simulink model "Nils_Bestehorn_WS19_modell"  (R2021b)
settings: Solver=FixedStepAuto  StartTime=0.0  StopTime=1  FixedStep=0.001  RelTol=1e-3
values from neighbouring files (symbols this model uses):
  c = 50    [Nils_Bestehorn_WS19_mfile.m]
  d = 0.05    [Nils_Bestehorn_WS19_mfile.m]
  dL = 5*exp(-6)    [Nils_Bestehorn_WS19_mfile.m]
  dM = 1.0*exp(-5)    [Nils_Bestehorn_WS19_mfile.m]
  JL = 2*exp(-5)    [Nils_Bestehorn_WS19_mfile.m]
  JM = 0.125*exp(-5)    [Nils_Bestehorn_WS19_mfile.m]
  LM = 1.0*exp(-3)    [Nils_Bestehorn_WS19_mfile.m]
  ML = 0.25    [Nils_Bestehorn_WS19_mfile.m]
  omegaL = 2.6*exp(-2)    [Nils_Bestehorn_WS19_mfile.m]
  omegaM = 0.1125    [Nils_Bestehorn_WS19_mfile.m]
  rL = 50*10^(-3)    (= 0.05)    [Nils_Bestehorn_WS19_mfile.m]
  RM = 1.5    [Nils_Bestehorn_WS19_mfile.m]
  rM = 25*10^(-3)    (= 0.025)    [Nils_Bestehorn_WS19_mfile.m]
  Uq = 24    [Nils_Bestehorn_WS19_mfile.m]
settings Model: Creator=nilsb  LastModifiedBy=nilsb

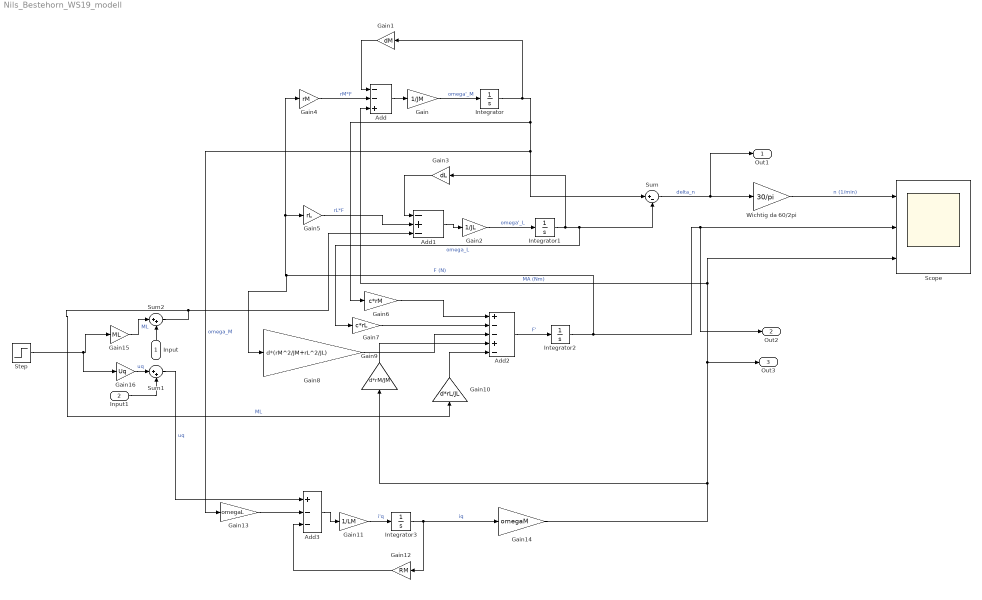
== system Nils_Bestehorn_WS19_modell ==
  Input : Inport
  Input1 : Inport  Port=2
  Add : Sum  Inputs=--+
  Add1 : Sum  Inputs=-+-
  Add2 : Sum  Inputs=+--+-
  Add3 : Sum  Inputs=+--
  Gain : Gain  Gain=1/JM
  Gain1 : Gain  Gain=dM
  Gain10 : Gain  Gain=d*rL/JL
  Gain11 : Gain  Gain=1/LM
  Gain12 : Gain  Gain=RM
  Gain13 : Gain  Gain=omegaL
  Gain14 : Gain  Gain=omegaM
  Gain15 : Gain  Gain=ML
  Gain16 : Gain  Gain=Uq
  Gain2 : Gain  Gain=1/JL
  Gain3 : Gain  Gain=dL
  Gain4 : Gain  Gain=rM
  Gain5 : Gain  Gain=rL
  Gain6 : Gain  Gain=c*rM
  Gain7 : Gain  Gain=c*rL
  Gain8 : Gain  Gain=d*(rM^2/JM+rL^2/JL)
  Gain9 : Gain  Gain=d*rM/JM
  Integrator{,1..3} (4 alike) : Integrator
  Scope : Scope  NumInputPorts=3
  Step : Step  Time=0.1  SampleTime=0
  Sum : Sum  Inputs=|+-
  Sum1 : Sum  Inputs=|++
  Sum2 : Sum  Inputs=|++
  Wichtig da 60/2pi : Gain  Gain=30/pi
  Out1 : Outport
  Out2 : Outport  Port=2
  Out3 : Outport  Port=3
  wires:
  Integrator/1 -> Gain1/1, Gain13/1, Sum/1, Gain6/1  "omega_M"
  Gain/1 -> Integrator/1  "omega'_M"
  Integrator1/1 -> Sum/2, Gain7/1, Gain3/1  "omega_L"
  Gain2/1 -> Integrator1/1  "omega'_L"
  Add/1 -> Gain/1
  Gain1/1 -> Add/1
  Gain4/1 -> Add/2  "rM*F"
  Gain14/1 -> Gain9/1, Add/3, Scope/3, Out3/1  "MA (Nm)"
  Add1/1 -> Gain2/1
  Gain3/1 -> Add1/1
  Gain5/1 -> Add1/2  "rL*F"
  Sum2/1 -> Gain10/1, Add1/3  "ML"
  Integrator2/1 -> Out2/1, Scope/2, Gain8/1, Gain4/1, Gain5/1  "F (N)"
  Add2/1 -> Integrator2/1  "F'"
  Gain6/1 -> Add2/1
  Gain7/1 -> Add2/2
  Gain8/1 -> Add2/3
  Gain9/1 -> Add2/4
  Gain10/1 -> Add2/5
  Sum/1 -> Out1/1, Wichtig da 60/2pi/1  "delta_n"
  Gain11/1 -> Integrator3/1  "i'q"
  Integrator3/1 -> Gain12/1, Gain14/1  "iq"
  Add3/1 -> Gain11/1
  Gain12/1 -> Add3/3
  Sum1/1 -> Add3/1  "uq"
  Gain13/1 -> Add3/2
  Step/1 -> Gain16/1, Gain15/1
  Gain15/1 -> Sum2/1  "ML"
  Input/1 -> Sum2/2
  Gain16/1 -> Sum1/1  "uq"
  Input1/1 -> Sum1/2
  Wichtig da 60/2pi/1 -> Scope/1  "n (1/min)"
